simulink model "Group30_SFWR_Assignment1_SIMULINK"  (R2022a)
settings: Solver=FixedStepAuto  StartTime=0.0  StopTime=10  FixedStep=1e-3  RelTol=1e-3  EnableMultiTasking=on
undefined symbols (not defined in the file): D0, D1, D10, D11, D12, D13, D2, D3, D4, D5, D6, D7, D8, D9, PTA0, PTA1, PTA2, PTB23, PTB9, PTC16, PTC17, PTC2, PTC3, PTC4, PTD0, PTD1, PTD2, PTD3
libraries: frdmk64flib x17, etargetslib x2
settings Model: ExtModeTrigDuration=5  Creator=ramu7  LastModifiedBy=scoob
settings OptimizationCC: EnhancedBackFolding=on  PassReuseOutputArgsAs=Individual arguments  ZeroExternalMemoryAtStartup=off  ZeroInternalMemoryAtStartup=off  MaxStackSize=64  OptimizeBlockOrder=speed  DifferentSizesBufferReuse=on  OptimizationCustomize=off  EfficientTunableParamExpr=on
settings DebuggingCC: ParameterTunabilityLossMsg=error
settings HardwareCC: ProdBitPerPointer=32  ProdBitPerSizeT=32  ProdBitPerPtrDiffT=32  ProdLargestAtomicInteger=Long  ProdLargestAtomicFloat=Double  ProdWordSize=32  ProdHWDeviceType=ARM Compatible->ARM Cortex
settings SFSimCC: MATLABDynamicMemAlloc=off
settings RTWCC: SystemTargetFile=ert.tlc  HardwareBoard=NXP FRDM-K64F  TLCOptions="-aInlineSetEventsForThisBaseRateFcn=TLC_FALSE -aSuppressMultiTaskScheduler=TLC_FALSE  -aRateBasedStepFcn=0"  TemplateMakefile=ert_default_tmf  Toolchain=GNU Tools for ARM Embedded Processors
settings CodeAppCC: ForceParamTrailComments=on  IgnoreCustomStorageClasses=off  OperatorAnnotations=on  SimulinkDataObjDesc=on  SFDataObjDesc=on  InsertBlockDesc=on
settings ERTTargetCC: ExtModeTransport=4  ExtModeMexFile=sendToCommService

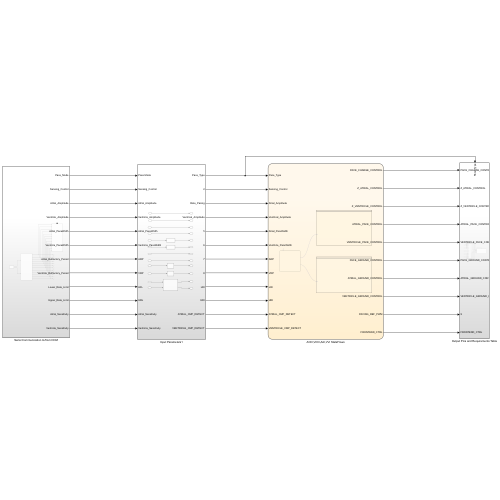
[thumbnail: Simulink's stored preview of the top-level diagram]
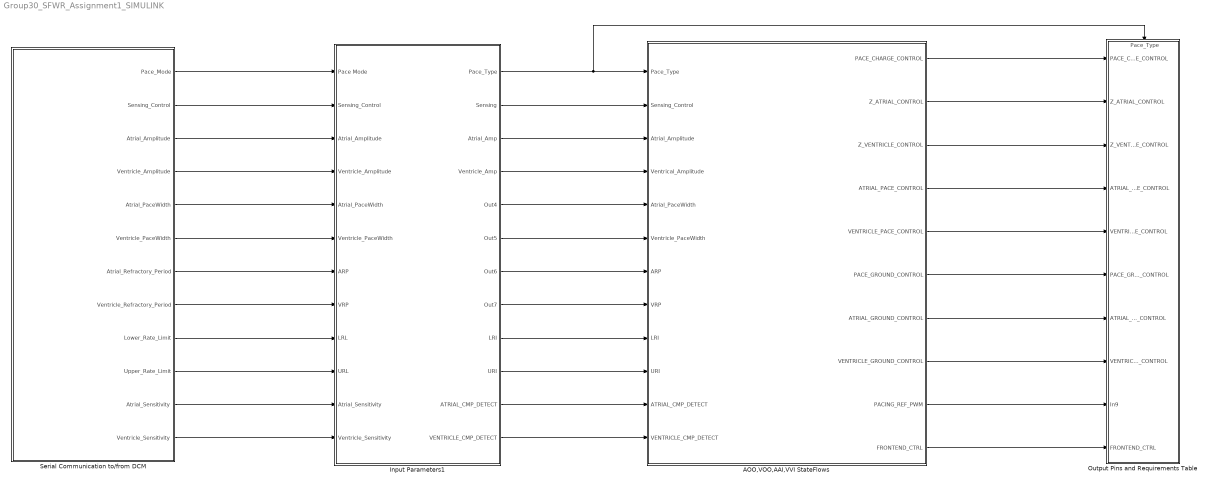
== system Group30_SFWR_Assignment1_SIMULINK ==
  AOO,VOO,AAI,VVI StateFlows : Stateflow chart  TreatAsAtomicUnit=on
      settings: PortSchema="{\"entries\":[{\"content\":{\"sides\":[{\"content\":{\"connectorIds\":[\"In1\",\"In9\",\"In2\",\"In10\",\"In11\",\"In12\",\"In8\",\"In7\",\"In5\",\"In6\",\"In3\",\"In4\"]},\"type\":\"ConnectorPlacement.EquallySpacedRectSide\",\"uuid\":\"9770646f-499d-4715-b3e0-54ec63e9a743\"},{\"content\":{\"connectorIds\":[\"Out1\",\"Out2\",\"Out3\",\"Out4\",\"Out5\",\"Out6\",\"Out7\",\"Out8\",\"Out9\",\"Out10\"],\"side\":\"RIGHT\"},\"type\":\"ConnectorPlacement.EquallySpacedRectSide\",\"uuid\":\"05a40026-c63e-4ef0-b71d-820a20f884f3\"},{\"content\":{\"connectorIds\":[],\"side\":\"TOP\"},\"type\":\"ConnectorPlacement.EquallySpacedRectSide\",\"uuid\":\"87d8712c-6353-4ad8-9661-243ca412d6bb\"}]},\"type\":\"ConnectorPlacement.EquallySpacedConnector\",\"uuid\":\"8262e7ac-98b5-44bf-add5-1ad3a0c707a1\"}],\"packageUris\":[\"http://schema.mathworks.com/mf0/Connector/R2020b\"],\"version\":\"1.0\"}"
  Input Parameters1 : Subsystem
  Output Pins and Requirements Table : Subsystem
      settings: PortSchema="{\"entries\":[{\"content\":{\"sides\":[{\"content\":{\"connectorIds\":[\"In1\",\"In2\",\"In3\",\"In4\",\"In5\",\"In6\",\"In7\",\"In8\",\"In9\",\"In10\"]},\"type\":\"ConnectorPlacement.EquallySpacedRectSide\",\"uuid\":\"40db26f6-8e31-4589-a315-6eea3b6d58f2\"},{\"content\":{\"connectorIds\":[],\"side\":\"RIGHT\"},\"type\":\"ConnectorPlacement.EquallySpacedRectSide\",\"uuid\":\"a6caef76-430e-44a7-94fa-313885a27199\"},{\"content\":{\"connectorIds\":[\"In11\"],\"side\":\"TOP\"},\"type\":\"ConnectorPlacement.EquallySpacedRectSide\",\"uuid\":\"9adbd5f8-a295-4590-a052-0a7aa200e456\"}]},\"type\":\"ConnectorPlacement.EquallySpacedConnector\",\"uuid\":\"6d560563-586d-4d61-8602-6a07324ae70c\"}],\"packageUris\":[\"http://schema.mathworks.com/mf0/Connector/R2020b\"],\"version\":\"1.0\"}"
  Serial Communication to/from DCM : Subsystem
  wires:
  AOO,VOO,AAI,VVI StateFlows/10(FRONTEND_CTRL) -> Output Pins and Requirements Table/10(FRONTEND_CTRL)
  AOO,VOO,AAI,VVI StateFlows/6(PACE_GROUND_CONTROL) -> Output Pins and Requirements Table/6(PACE_GROUND_CONTROL)
  AOO,VOO,AAI,VVI StateFlows/2(Z_ATRIAL_CONTROL) -> Output Pins and Requirements Table/2(Z_ATRIAL_CONTROL)
  AOO,VOO,AAI,VVI StateFlows/3(Z_VENTRICLE_CONTROL) -> Output Pins and Requirements Table/3(Z_VENTRICLE_CONTROL)
  AOO,VOO,AAI,VVI StateFlows/1(PACE_CHARGE_CONTROL) -> Output Pins and Requirements Table/1(PACE_CHARGE_CONTROL)
  AOO,VOO,AAI,VVI StateFlows/4(ATRIAL_PACE_CONTROL) -> Output Pins and Requirements Table/4(ATRIAL_PACE_CONTROL)
  AOO,VOO,AAI,VVI StateFlows/9(PACING_REF_PWM) -> Output Pins and Requirements Table/9(In9)
  AOO,VOO,AAI,VVI StateFlows/7(ATRIAL_GROUND_CONTROL) -> Output Pins and Requirements Table/7(ATRIAL_GROUND_CONTROL)
  AOO,VOO,AAI,VVI StateFlows/5(VENTRICLE_PACE_CONTROL) -> Output Pins and Requirements Table/5(VENTRICLE_PACE_CONTROL)
  AOO,VOO,AAI,VVI StateFlows/8(VENTRICLE_GROUND_CONTROL) -> Output Pins and Requirements Table/8(VENTRICLE_GROUND_CONTROL)
  Input Parameters1/1(Pace_Type) -> Output Pins and Requirements Table/11(Pace_Type), AOO,VOO,AAI,VVI StateFlows/1(Pace_Type)
  Input Parameters1/2(Sensing) -> AOO,VOO,AAI,VVI StateFlows/9(Sensing_Control)
  Input Parameters1/3(Atrial_Amp) -> AOO,VOO,AAI,VVI StateFlows/2(Atrial_Amplitude)
  Input Parameters1/4(Ventricle_Amp) -> AOO,VOO,AAI,VVI StateFlows/10(Ventrical_Amplitude)
  Input Parameters1/6(Out5) -> AOO,VOO,AAI,VVI StateFlows/12(Ventricle_PaceWidth)
  Input Parameters1/5(Out4) -> AOO,VOO,AAI,VVI StateFlows/11(Atrial_PaceWidth)
  Input Parameters1/7(Out6) -> AOO,VOO,AAI,VVI StateFlows/8(ARP)
  Input Parameters1/8(Out7) -> AOO,VOO,AAI,VVI StateFlows/7(VRP)
  Input Parameters1/9(LRI) -> AOO,VOO,AAI,VVI StateFlows/5(LRI)
  Input Parameters1/10(URI) -> AOO,VOO,AAI,VVI StateFlows/6(URI)
  Input Parameters1/11(ATRIAL_CMP_DETECT) -> AOO,VOO,AAI,VVI StateFlows/3(ATRIAL_CMP_DETECT)
  Input Parameters1/12(VENTRICLE_CMP_DETECT) -> AOO,VOO,AAI,VVI StateFlows/4(VENTRICLE_CMP_DETECT)
  Serial Communication to/from DCM/1(Pace_Mode) -> Input Parameters1/1(Pace Mode)
  Serial Communication to/from DCM/2(Sensing_Control) -> Input Parameters1/2(Sensing_Control)
  Serial Communication to/from DCM/3(Atrial_Amplitude) -> Input Parameters1/3(Atrial_Amplitude)
  Serial Communication to/from DCM/4(Ventricle_Amplitude) -> Input Parameters1/4(Ventricle_Amplitude)
  Serial Communication to/from DCM/5(Atrial_PaceWidth) -> Input Parameters1/5(Atrial_PaceWidth)
  Serial Communication to/from DCM/6(Ventricle_PaceWidth) -> Input Parameters1/6(Ventricle_PaceWidth)
  Serial Communication to/from DCM/7(Atrial_Refractory_Period) -> Input Parameters1/7(ARP)
  Serial Communication to/from DCM/8(Ventricle_Refractory_Period) -> Input Parameters1/8(VRP)
  Serial Communication to/from DCM/9(Lower_Rate_Limit) -> Input Parameters1/9(LRL)
  Serial Communication to/from DCM/10(Upper_Rate_Limit) -> Input Parameters1/10(URL)
  Serial Communication to/from DCM/11(Atrial_Sensitivity) -> Input Parameters1/11(Atrial_Sensitivity)
  Serial Communication to/from DCM/12(Ventricle_Sensitivity) -> Input Parameters1/12(Ventricle_Sensitivity)

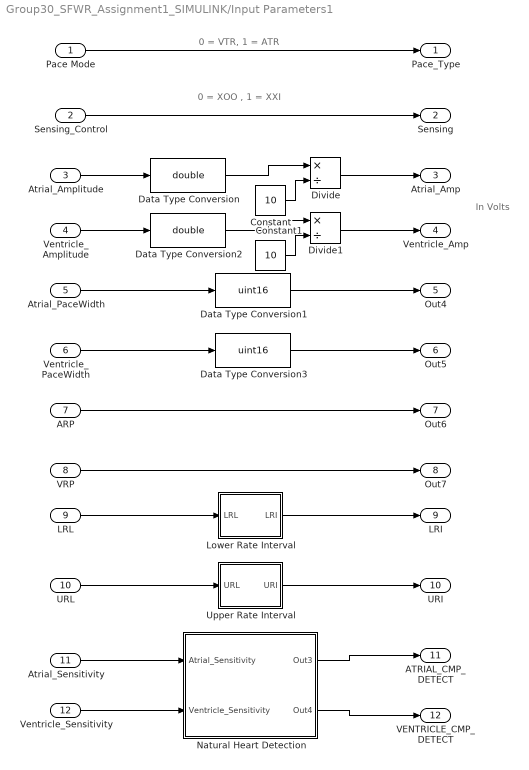
== system Group30_SFWR_Assignment1_SIMULINK/Input Parameters1 ==
  note: In Volts
  note: 0 = XOO , 1 = XXI
  note: 0 = VTR, 1 = ATR
  Pace Mode : Inport  OutDataTypeStr=uint8
  Sensing_Control : Inport  Port=2  OutDataTypeStr=uint8
  Atrial_Amplitude : Inport  Port=3  OutDataTypeStr=uint8
  Ventricle_Amplitude : Inport  Port=4  OutDataTypeStr=uint8
  Atrial_PaceWidth : Inport  Port=5  OutDataTypeStr=uint8
  Ventricle_PaceWidth : Inport  Port=6  OutDataTypeStr=uint8
  ARP : Inport  Port=7  OutDataTypeStr=uint16
  VRP : Inport  Port=8  OutDataTypeStr=uint16
  LRL : Inport  Port=9  OutDataTypeStr=uint8
  URL : Inport  Port=10
  Atrial_Sensitivity : Inport  Port=11  OutDataTypeStr=uint8
  Ventricle_Sensitivity : Inport  Port=12  OutDataTypeStr=uint8
  Constant : Constant  Value=10
  Constant1 : Constant  Value=10
  Data Type Conversion : DataTypeConversion  OutDataTypeStr=double  SaturateOnIntegerOverflow=off  RndMeth=Floor
  Data Type Conversion1 : DataTypeConversion  OutDataTypeStr=uint16  SaturateOnIntegerOverflow=off  RndMeth=Floor
  Data Type Conversion2 : DataTypeConversion  OutDataTypeStr=double  SaturateOnIntegerOverflow=off  RndMeth=Floor
  Data Type Conversion3 : DataTypeConversion  OutDataTypeStr=uint16  SaturateOnIntegerOverflow=off  RndMeth=Floor
  Divide : Product  Inputs=*/
  Divide1 : Product  Inputs=*/
  Lower Rate Interval : Subsystem
  Natural Heart Detection : Subsystem
  Upper Rate Interval : Subsystem
  Pace_Type : Outport
  Sensing : Outport  Port=2
  Atrial_Amp : Outport  Port=3
  Ventricle_Amp : Outport  Port=4
  Out4 : Outport  Port=5
  Out5 : Outport  Port=6
  Out6 : Outport  Port=7
  Out7 : Outport  Port=8
  LRI : Outport  Port=9
  URI : Outport  Port=10
  ATRIAL_CMP_DETECT : Outport  Port=11
  VENTRICLE_CMP_DETECT : Outport  Port=12
  wires:
  Ventricle_PaceWidth/1 -> Data Type Conversion3/1
  VRP/1 -> Out7/1
  Atrial_PaceWidth/1 -> Data Type Conversion1/1
  Sensing_Control/1 -> Sensing/1
  ARP/1 -> Out6/1
  Pace Mode/1 -> Pace_Type/1
  Lower Rate Interval/1(LRI) -> LRI/1
  Upper Rate Interval/1(URI) -> URI/1
  Natural Heart Detection/1(Out3) -> ATRIAL_CMP_DETECT/1
  Natural Heart Detection/2(Out4) -> VENTRICLE_CMP_DETECT/1
  LRL/1 -> Lower Rate Interval/1(LRL)
  URL/1 -> Upper Rate Interval/1(URL)
  Atrial_Sensitivity/1 -> Natural Heart Detection/1(Atrial_Sensitivity)
  Ventricle_Sensitivity/1 -> Natural Heart Detection/2(Ventricle_Sensitivity)
  Data Type Conversion3/1 -> Out5/1
  Data Type Conversion1/1 -> Out4/1
  Atrial_Amplitude/1 -> Data Type Conversion/1
  Data Type Conversion/1 -> Divide/1
  Constant/1 -> Divide/2
  Divide/1 -> Atrial_Amp/1
  Constant1/1 -> Divide1/2
  Data Type Conversion2/1 -> Divide1/1
  Ventricle_Amplitude/1 -> Data Type Conversion2/1
  Divide1/1 -> Ventricle_Amp/1

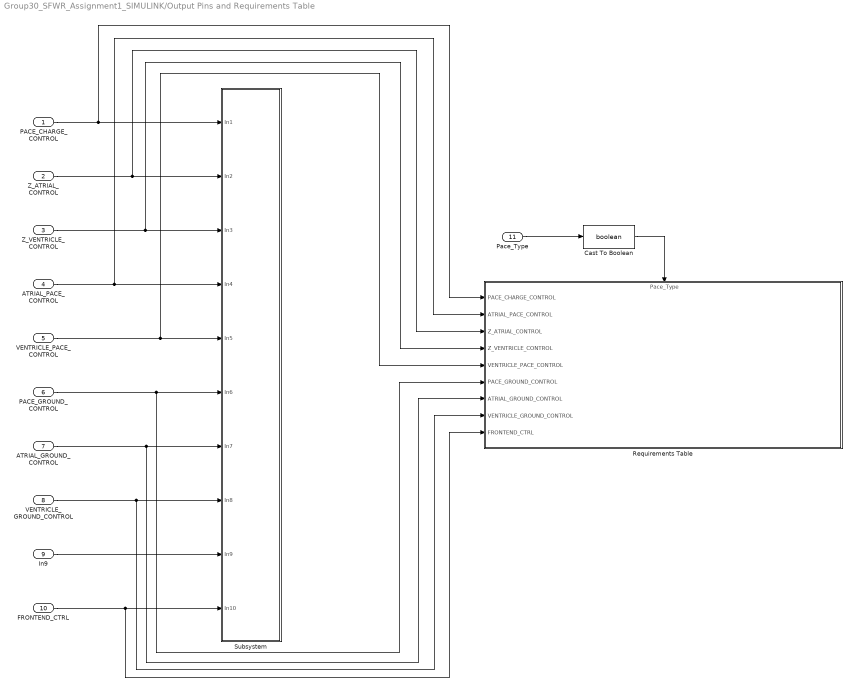
== system Group30_SFWR_Assignment1_SIMULINK/Output Pins and Requirements Table ==
  PACE_CHARGE_CONTROL : Inport
  Z_ATRIAL_CONTROL : Inport  Port=2
  Z_VENTRICLE_CONTROL : Inport  Port=3
  ATRIAL_PACE_CONTROL : Inport  Port=4
  VENTRICLE_PACE_CONTROL : Inport  Port=5
  PACE_GROUND_CONTROL : Inport  Port=6
  ATRIAL_GROUND_CONTROL : Inport  Port=7
  VENTRICLE_GROUND_CONTROL : Inport  Port=8
  In9 : Inport  Port=9
  FRONTEND_CTRL : Inport  Port=10
  Pace_Type : Inport  Port=11
  Cast To Boolean : DataTypeConversion  OutDataTypeStr=boolean  SaturateOnIntegerOverflow=off  RndMeth=Floor
  Requirements Table : Subsystem
      settings: PortSchema="{\"entries\":[{\"content\":{\"sides\":[{\"content\":{\"connectorIds\":[\"In1\",\"In2\",\"In3\",\"In4\",\"In5\",\"In6\",\"In7\",\"In8\",\"In9\"]},\"type\":\"ConnectorPlacement.EquallySpacedRectSide\",\"uuid\":\"46327938-4478-40d2-aac6-72547228615e\"},{\"content\":{\"connectorIds\":[],\"side\":\"RIGHT\"},\"type\":\"ConnectorPlacement.EquallySpacedRectSide\",\"uuid\":\"a4c12f67-beb4-4537-be9d-262931108289\"},{\"content\":{\"connectorIds\":[\"In10\"],\"side\":\"TOP\"},\"type\":\"ConnectorPlacement.EquallySpacedRectSide\",\"uuid\":\"a653f2ff-3266-45dd-85b5-df796fc313fd\"}]},\"type\":\"ConnectorPlacement.EquallySpacedConnector\",\"uuid\":\"ede91063-bb98-4867-a1df-25b64c24a60e\"}],\"packageUris\":[\"http://schema.mathworks.com/mf0/Connector/R2020b\"],\"version\":\"1.0\"}"
  Subsystem : Subsystem
  wires:
  Pace_Type/1 -> Cast To Boolean/1
  PACE_CHARGE_CONTROL/1 -> Requirements Table/1(PACE_CHARGE_CONTROL), Subsystem/1(In1)
  Z_ATRIAL_CONTROL/1 -> Requirements Table/3(Z_ATRIAL_CONTROL), Subsystem/2(In2)
  Z_VENTRICLE_CONTROL/1 -> Requirements Table/4(Z_VENTRICLE_CONTROL), Subsystem/3(In3)
  ATRIAL_PACE_CONTROL/1 -> Requirements Table/2(ATRIAL_PACE_CONTROL), Subsystem/4(In4)
  VENTRICLE_PACE_CONTROL/1 -> Requirements Table/5(VENTRICLE_PACE_CONTROL), Subsystem/5(In5)
  PACE_GROUND_CONTROL/1 -> Requirements Table/6(PACE_GROUND_CONTROL), Subsystem/6(In6)
  ATRIAL_GROUND_CONTROL/1 -> Requirements Table/7(ATRIAL_GROUND_CONTROL), Subsystem/7(In7)
  VENTRICLE_GROUND_CONTROL/1 -> Subsystem/8(In8), Requirements Table/8(VENTRICLE_GROUND_CONTROL)
  In9/1 -> Subsystem/9(In9)
  FRONTEND_CTRL/1 -> Subsystem/10(In10), Requirements Table/9(FRONTEND_CTRL)
  Cast To Boolean/1 -> Requirements Table/10(Pace_Type)

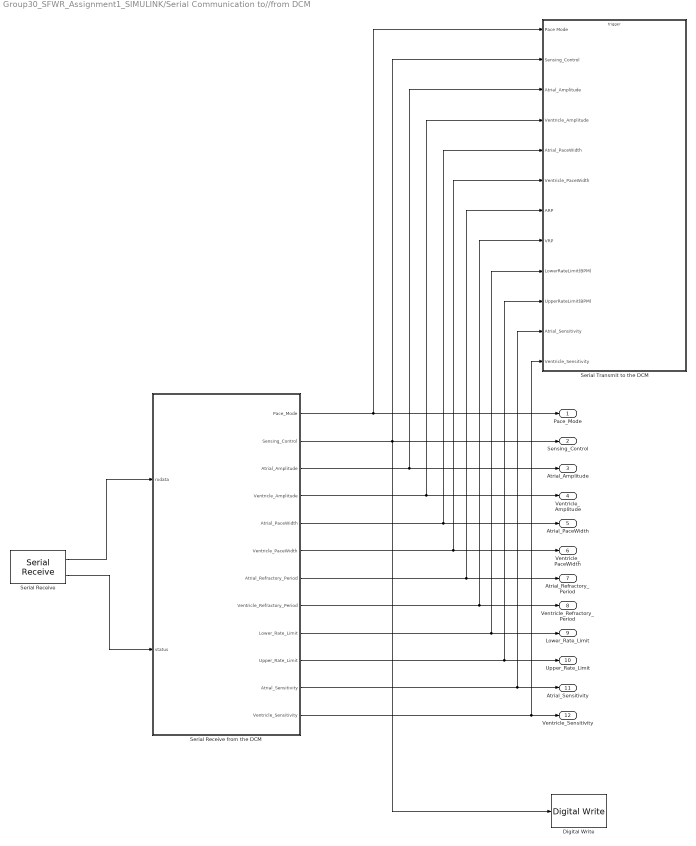
== system Group30_SFWR_Assignment1_SIMULINK/Serial Communication to//from DCM ==
  Digital Write : frdmk64flib/Digital Write  Whichpin=BLUE_LED
  Serial Receive : frdmk64flib/Serial Receive  SCIModule=0  Baudrate=uint32(9600)  Parity=None  StopBits=1  HardwareFlowControl=None  ByteOrder=LittleEndian  DataType=uint8  DataLength=16  BlockingMode=off  OutputStatus=on  SampleTime=-1
  Serial Receive from the DCM : Stateflow chart  TreatAsAtomicUnit=on
      settings: PortSchema="{\"entries\":[{\"content\":{\"sides\":[{\"content\":{\"connectorIds\":[\"In1\",\"In2\"]},\"type\":\"ConnectorPlacement.EquallySpacedRectSide\",\"uuid\":\"2959f4f4-8806-48ae-afb0-f3f6f5a900bd\"},{\"content\":{\"connectorIds\":[\"Out6\",\"Out7\",\"Out1\",\"Out9\",\"Out2\",\"Out10\",\"Out3\",\"Out11\",\"Out5\",\"Out8\",\"Out4\",\"Out12\"],\"side\":\"RIGHT\"},\"type\":\"ConnectorPlacement.EquallySpacedRectSide\",\"uuid\":\"cafcb0cc-74e9-4bf6-9034-07be9eddf5a8\"},{\"content\":{\"connectorIds\":[],\"side\":\"TOP\"},\"type\":\"ConnectorPlacement.EquallySpacedRectSide\",\"uuid\":\"46ea3eb1-522e-47a6-9d77-75fe2cddba2b\"}]},\"type\":\"ConnectorPlacement.EquallySpacedConnector\",\"uuid\":\"dcbaec72-729d-430b-8c38-c6d2009603d6\"}],\"packageUris\":[\"http://schema.mathworks.com/mf0/Connector/R2020b\"],\"version\":\"1.0\"}"
  Serial Transmit to the DCM : Subsystem
  Pace_Mode : Outport
  Sensing_Control : Outport  Port=2
  Atrial_Amplitude : Outport  Port=3
  Ventricle_Amplitude : Outport  Port=4
  Atrial_PaceWidth : Outport  Port=5
  Ventricle_PaceWidth : Outport  Port=6
  Atrial_Refractory_Period : Outport  Port=7
  Ventricle_Refractory_Period : Outport  Port=8
  Lower_Rate_Limit : Outport  Port=9
  Upper_Rate_Limit : Outport  Port=10
  Atrial_Sensitivity : Outport  Port=11
  Ventricle_Sensitivity : Outport  Port=12
  wires:
  Serial Receive from the DCM/8(Upper_Rate_Limit) -> Upper_Rate_Limit/1, Serial Transmit to the DCM/10(UpperRateLimit(BPM))
  Serial Receive from the DCM/11(Ventricle_Refractory_Period) -> Ventricle_Refractory_Period/1, Serial Transmit to the DCM/8(VRP)
  Serial Receive from the DCM/5(Lower_Rate_Limit) -> Lower_Rate_Limit/1, Serial Transmit to the DCM/9(LowerRateLimit(BPM))
  Serial Receive from the DCM/10(Ventricle_PaceWidth) -> Ventricle_PaceWidth/1, Serial Transmit to the DCM/6(Ventricle_PaceWidth)
  Serial Receive from the DCM/6(Pace_Mode) -> Pace_Mode/1, Serial Transmit to the DCM/1(Pace Mode)
  Serial Receive from the DCM/2(Atrial_PaceWidth) -> Atrial_PaceWidth/1, Serial Transmit to the DCM/5(Atrial_PaceWidth)
  Serial Receive from the DCM/4(Atrial_Sensitivity) -> Atrial_Sensitivity/1, Serial Transmit to the DCM/11(Atrial_Sensitivity)
  Serial Receive from the DCM/7(Sensing_Control) -> Digital Write/1, Sensing_Control/1, Serial Transmit to the DCM/2(Sensing_Control)
  Serial Receive from the DCM/1(Atrial_Amplitude) -> Atrial_Amplitude/1, Serial Transmit to the DCM/3(Atrial_Amplitude)
  Serial Receive from the DCM/9(Ventricle_Amplitude) -> Ventricle_Amplitude/1, Serial Transmit to the DCM/4(Ventricle_Amplitude)
  Serial Receive from the DCM/3(Atrial_Refractory_Period) -> Atrial_Refractory_Period/1, Serial Transmit to the DCM/7(ARP)
  Serial Receive from the DCM/12(Ventricle_Sensitivity) -> Ventricle_Sensitivity/1, Serial Transmit to the DCM/12(Ventricle_Sensitivity)
  Serial Receive/1 -> Serial Receive from the DCM/1(rxdata)
  Serial Receive/2 -> Serial Receive from the DCM/2(status)

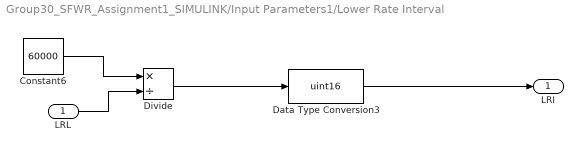
== system Group30_SFWR_Assignment1_SIMULINK/Input Parameters1/Lower Rate Interval ==
  LRL : Inport
  Constant6 : Constant  Value=60000
  Data Type Conversion3 : DataTypeConversion  OutDataTypeStr=uint16  SaturateOnIntegerOverflow=off  RndMeth=Floor
  Divide : Product  Inputs=*/
  LRI : Outport
  wires:
  Constant6/1 -> Divide/1
  LRL/1 -> Divide/2
  Divide/1 -> Data Type Conversion3/1
  Data Type Conversion3/1 -> LRI/1

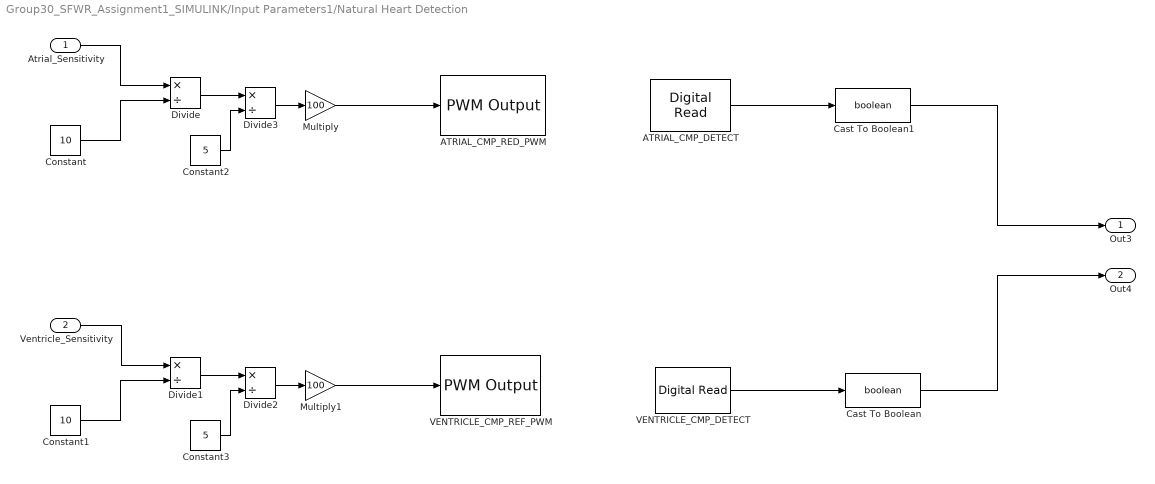
== system Group30_SFWR_Assignment1_SIMULINK/Input Parameters1/Natural Heart Detection ==
  Atrial_Sensitivity : Inport
  Ventricle_Sensitivity : Inport  Port=2
  ATRIAL_CMP_DETECT : frdmk64flib/Digital Read  Whichpin=PTC16 (D0)  SampleTime=-1
  ATRIAL_CMP_RED_PWM : frdmk64flib/PWM Output  Whichpin=PTC2 (D6)  InitialFrequency=2000  InitialDutyCycle=51
  Cast To Boolean : DataTypeConversion  OutDataTypeStr=boolean  SaturateOnIntegerOverflow=off  RndMeth=Floor
  Cast To Boolean1 : DataTypeConversion  OutDataTypeStr=boolean  SaturateOnIntegerOverflow=off  RndMeth=Floor
  Constant : Constant  Value=10
  Constant1 : Constant  Value=10
  Constant2 : Constant  Value=5
  Constant3 : Constant  Value=5
  Divide{,1..3} (4 alike) : Product  Inputs=*/
  Multiply : Gain  Gain=100
  Multiply1 : Gain  Gain=100
  VENTRICLE_CMP_DETECT : frdmk64flib/Digital Read  Whichpin=PTC17 (D1)  SampleTime=-1
  VENTRICLE_CMP_REF_PWM : frdmk64flib/PWM Output  Whichpin=PTA1 (D3)  InitialFrequency=2000  InitialDutyCycle=60
  Out3 : Outport
  Out4 : Outport  Port=2
  wires:
  Multiply1/1 -> VENTRICLE_CMP_REF_PWM/1
  Multiply/1 -> ATRIAL_CMP_RED_PWM/1
  VENTRICLE_CMP_DETECT/1 -> Cast To Boolean/1
  ATRIAL_CMP_DETECT/1 -> Cast To Boolean1/1
  Cast To Boolean1/1 -> Out3/1
  Cast To Boolean/1 -> Out4/1
  Atrial_Sensitivity/1 -> Divide/1
  Constant/1 -> Divide/2
  Constant1/1 -> Divide1/2
  Ventricle_Sensitivity/1 -> Divide1/1
  Divide1/1 -> Divide2/1
  Divide/1 -> Divide3/1
  Constant2/1 -> Divide3/2
  Constant3/1 -> Divide2/2
  Divide3/1 -> Multiply/1
  Divide2/1 -> Multiply1/1

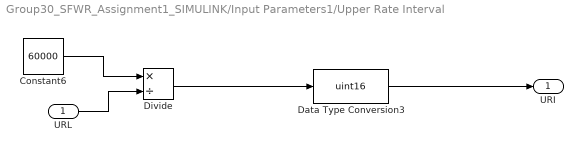
== system Group30_SFWR_Assignment1_SIMULINK/Input Parameters1/Upper Rate Interval ==
  URL : Inport
  Constant6 : Constant  Value=60000
  Data Type Conversion3 : DataTypeConversion  OutDataTypeStr=uint16  SaturateOnIntegerOverflow=off  RndMeth=Floor
  Divide : Product  Inputs=*/
  URI : Outport
  wires:
  Divide/1 -> Data Type Conversion3/1
  URL/1 -> Divide/2
  Constant6/1 -> Divide/1
  Data Type Conversion3/1 -> URI/1

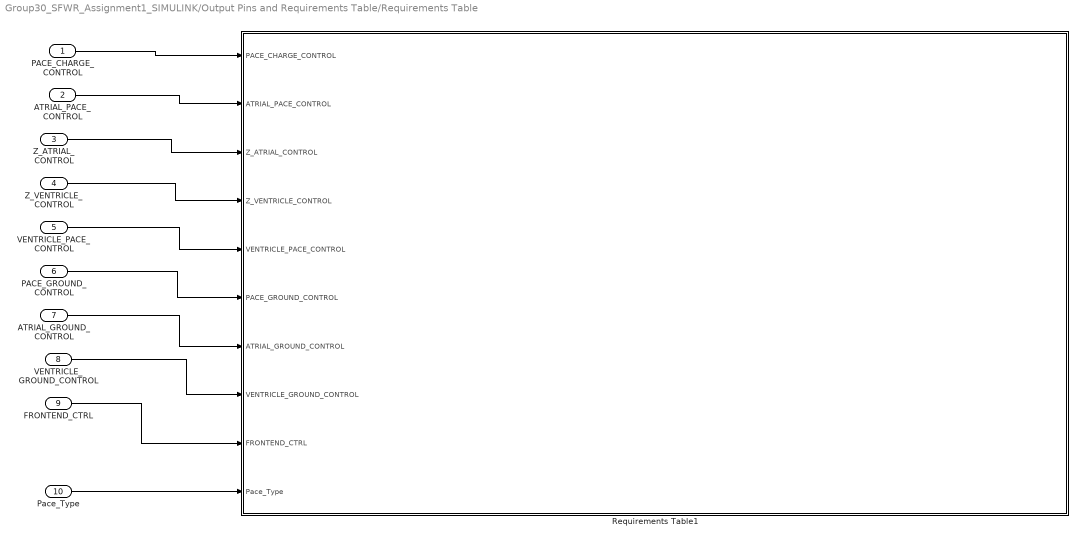
== system Group30_SFWR_Assignment1_SIMULINK/Output Pins and Requirements Table/Requirements Table ==
  PACE_CHARGE_CONTROL : Inport
  ATRIAL_PACE_CONTROL : Inport  Port=2
  Z_ATRIAL_CONTROL : Inport  Port=3
  Z_VENTRICLE_CONTROL : Inport  Port=4
  VENTRICLE_PACE_CONTROL : Inport  Port=5
  PACE_GROUND_CONTROL : Inport  Port=6
  ATRIAL_GROUND_CONTROL : Inport  Port=7
  VENTRICLE_GROUND_CONTROL : Inport  Port=8
  FRONTEND_CTRL : Inport  Port=9
  Pace_Type : Inport  Port=10
  Requirements Table1 : Requirements Table  TreatAsAtomicUnit=on
  wires:
  PACE_CHARGE_CONTROL/1 -> Requirements Table1/1(PACE_CHARGE_CONTROL)
  ATRIAL_PACE_CONTROL/1 -> Requirements Table1/2(ATRIAL_PACE_CONTROL)
  Z_ATRIAL_CONTROL/1 -> Requirements Table1/3(Z_ATRIAL_CONTROL)
  Z_VENTRICLE_CONTROL/1 -> Requirements Table1/4(Z_VENTRICLE_CONTROL)
  VENTRICLE_PACE_CONTROL/1 -> Requirements Table1/5(VENTRICLE_PACE_CONTROL)
  PACE_GROUND_CONTROL/1 -> Requirements Table1/6(PACE_GROUND_CONTROL)
  ATRIAL_GROUND_CONTROL/1 -> Requirements Table1/7(ATRIAL_GROUND_CONTROL)
  VENTRICLE_GROUND_CONTROL/1 -> Requirements Table1/8(VENTRICLE_GROUND_CONTROL)
  FRONTEND_CTRL/1 -> Requirements Table1/9(FRONTEND_CTRL)
  Pace_Type/1 -> Requirements Table1/10(Pace_Type)

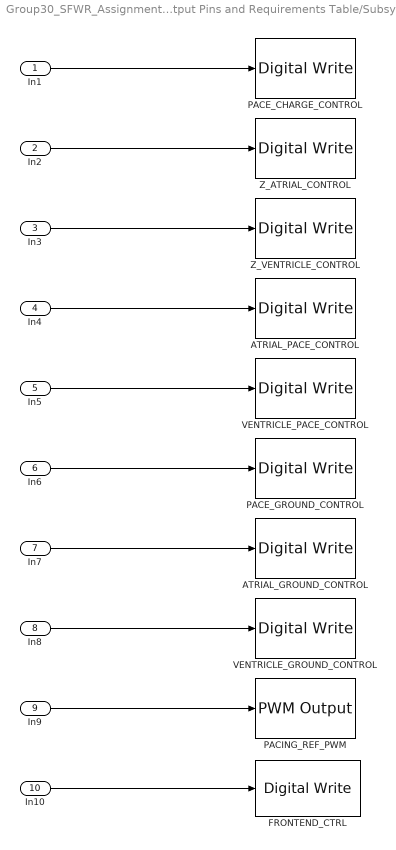
== system Group30_SFWR_Assignment1_SIMULINK/Output Pins and Requirements Table/Subsystem ==
  In1 : Inport
  In2 : Inport  Port=2
  In3 : Inport  Port=3
  In4 : Inport  Port=4
  In5 : Inport  Port=5
  In6 : Inport  Port=6
  In7 : Inport  Port=7
  In8 : Inport  Port=8
  In9 : Inport  Port=9
  In10 : Inport  Port=10
  ATRIAL_GROUND_CONTROL : frdmk64flib/Digital Write  Whichpin=PTD2 (D11)
  ATRIAL_PACE_CONTROL : frdmk64flib/Digital Write  Whichpin=PTA0 (D8)
  FRONTEND_CTRL : frdmk64flib/Digital Write  Whichpin=PTD1 (D13)
  PACE_CHARGE_CONTROL : frdmk64flib/Digital Write  Whichpin=PTB9 (D2)
  PACE_GROUND_CONTROL : frdmk64flib/Digital Write  Whichpin=PTD0 (D10)
  PACING_REF_PWM : frdmk64flib/PWM Output  Whichpin=PTA2 (D5)  InitialFrequency=2000  InitialDutyCycle=40
  VENTRICLE_GROUND_CONTROL : frdmk64flib/Digital Write  Whichpin=PTD3 (D12)
  VENTRICLE_PACE_CONTROL : frdmk64flib/Digital Write  Whichpin=PTC4 (D9)
  Z_ATRIAL_CONTROL : frdmk64flib/Digital Write  Whichpin=PTB23 (D4)
  Z_VENTRICLE_CONTROL : frdmk64flib/Digital Write  Whichpin=PTC3 (D7)
  wires:
  In5/1 -> VENTRICLE_PACE_CONTROL/1
  In9/1 -> PACING_REF_PWM/1
  In7/1 -> ATRIAL_GROUND_CONTROL/1
  In10/1 -> FRONTEND_CTRL/1
  In1/1 -> PACE_CHARGE_CONTROL/1
  In6/1 -> PACE_GROUND_CONTROL/1
  In4/1 -> ATRIAL_PACE_CONTROL/1
  In2/1 -> Z_ATRIAL_CONTROL/1
  In3/1 -> Z_VENTRICLE_CONTROL/1
  In8/1 -> VENTRICLE_GROUND_CONTROL/1

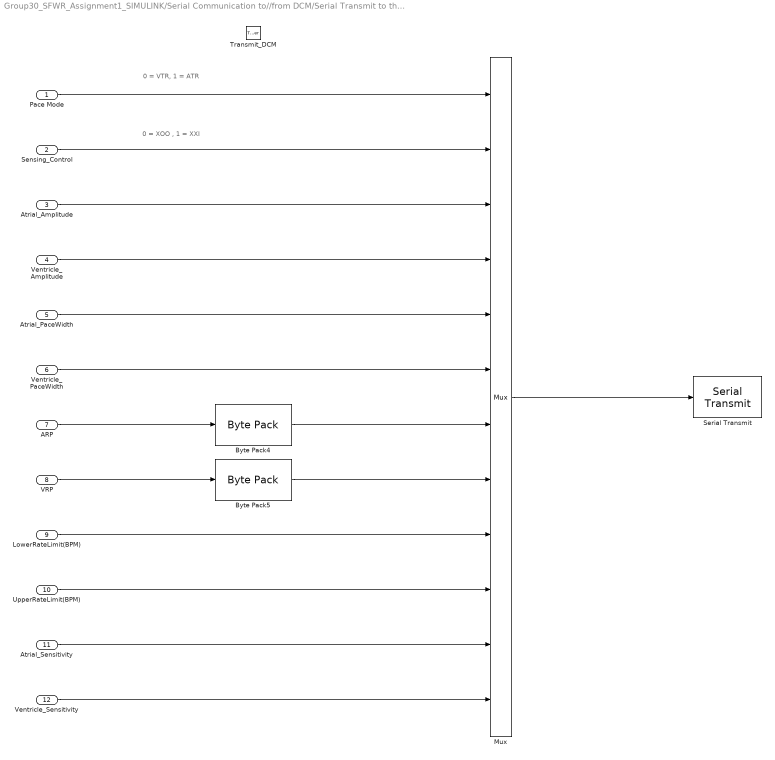
== system Group30_SFWR_Assignment1_SIMULINK/Serial Communication to//from DCM/Serial Transmit to the DCM ==
  note: 0 = VTR, 1 = ATR
  note: 0 = XOO , 1 = XXI
  Pace Mode : Inport  OutDataTypeStr=uint8
  Sensing_Control : Inport  Port=2  OutDataTypeStr=uint8
  Atrial_Amplitude : Inport  Port=3  OutDataTypeStr=uint8
  Ventricle_Amplitude : Inport  Port=4  OutDataTypeStr=uint8
  Atrial_PaceWidth : Inport  Port=5  OutDataTypeStr=uint8
  Ventricle_PaceWidth : Inport  Port=6  OutDataTypeStr=uint8
  ARP : Inport  Port=7  OutDataTypeStr=uint16
  VRP : Inport  Port=8  OutDataTypeStr=uint16
  LowerRateLimit(BPM) : Inport  Port=9
  UpperRateLimit(BPM) : Inport  Port=10
  Atrial_Sensitivity : Inport  Port=11  OutDataTypeStr=uint8
  Ventricle_Sensitivity : Inport  Port=12  OutDataTypeStr=uint8
  Transmit_DCM : TriggerPort  TriggerType=function-call  IsSimulinkFunction=on  FunctionName=Transmit_DCM  VariantControl=Variant
  Byte Pack4 : etargetslib/Byte Pack  datatypes={'uint16'}  byteAlign=1
  Byte Pack5 : etargetslib/Byte Pack  datatypes={'uint16'}  byteAlign=1
  Mux : Mux  Inputs=12
  Serial Transmit : frdmk64flib/Serial Transmit  SCIModule=0  Baudrate=uint32(9600)  Parity=None  StopBits=1  HardwareFlowControl=None  ByteOrder=LittleEndian  BlockingMode=on  OutputStatus=off
  wires:
  Mux/1 -> Serial Transmit/1
  UpperRateLimit(BPM)/1 -> Mux/10
  VRP/1 -> Byte Pack5/1
  ARP/1 -> Byte Pack4/1
  Sensing_Control/1 -> Mux/2
  Pace Mode/1 -> Mux/1
  LowerRateLimit(BPM)/1 -> Mux/9
  Atrial_Amplitude/1 -> Mux/3
  Ventricle_Amplitude/1 -> Mux/4
  Atrial_PaceWidth/1 -> Mux/5
  Ventricle_PaceWidth/1 -> Mux/6
  Byte Pack4/1 -> Mux/7
  Byte Pack5/1 -> Mux/8
  Atrial_Sensitivity/1 -> Mux/11
  Ventricle_Sensitivity/1 -> Mux/12

== stateflow chart Group30_SFWR_Assignment1_SIMULINK/AOO,VOO,AAI,VVI StateFlows ==
  state VENTRICLE MODES (VOO and VVI) [group]
    state SENSE_Ventricle
    note: Heartbeat not found after the LRI period, pace the heart
    note: Heartbeat found, reset LRI
    state PACE_Charge_Ventricle
      %Charging C22 and discharing C21
      entry:
      PACING_REF_PWM = (10*Ventrical_Amplitude/5)
      PACE_CHARGE_CONTROL = true
      VENTRICLE_PACE_CONTROL = false
      VENTRICLE_GROUND_CONTROL=true
      ATRIAL_PACE_CONTROL =false
      ATRIAL_GROUND_CONTROL = false
      FRONTEND_CTRL = false
      PACE_GROUND_CONTROL = true
    state PACE_Discharge_Ventricle
      %Discharging C22
      entry:
      PACE_CHARGE_CONTROL = false
      VENTRICLE_PACE_CONTROL = true
      VENTRICLE_GROUND_CONTROL= false
      FRONTEND_CTRL = false
    SENSE_Ventricle -> PACE_Discharge_Ventricle [order 1] : after(LRI - VRP,msec) [VENTRICLE_CMP_DETECT == false]
    SENSE_Ventricle -> PACE_Charge_Ventricle [order 2] : [VENTRICLE_CMP_DETECT == true]
    PACE_Charge_Ventricle -> SENSE_Ventricle [order 1] : after(VRP,msec)[Sensing_Control == true]{FRONTEND_CTRL = true}
    PACE_Charge_Ventricle -> PACE_Discharge_Ventricle [order 2] : after(LRI - Ventricle_PaceWidth,msec)[Sensing_Control == false]
    PACE_Discharge_Ventricle -> PACE_Charge_Ventricle : after(Ventricle_PaceWidth,msec)
  state Default_State
    entry:
    FRONTEND_CTRL = false
    PACE_GROUND_CONTROL = false
    Z_ATRIAL_CONTROL = false
    Z_VENTRICLE_CONTROL = false
    PACE_CHARGE_CONTROL = false
    VENTRICLE_PACE_CONTROL = false
    VENTRICLE_GROUND_CONTROL = false
    ATRIAL_PACE_CONTROL = false
    ATRIAL_GROUND_CONTROL = false
  state ATRIAL MODES (AOO and AAI) [group]
    state SENSE_Atrial
    note: Heartbeat not found after the LRI period, pace the heart
    note: Heartbeat found, reset LRI
    state PACE_Charge_Atrial
      %Charging C22 and discharing C21
      entry:
      PACING_REF_PWM = (10*Atrial_Amplitude/5)
      PACE_CHARGE_CONTROL = true
      VENTRICLE_PACE_CONTROL = false
      VENTRICLE_GROUND_CONTROL=false
      ATRIAL_PACE_CONTROL =false
      ATRIAL_GROUND_CONTROL = true
      FRONTEND_CTRL = false
      PACE_GROUND_CONTROL = true
    state PACE_Discharge_Atrial
      %Discharging C22
      entry:
      PACE_CHARGE_CONTROL = false
      ATRIAL_PACE_CONTROL = true
      ATRIAL_GROUND_CONTROL = false
      FRONTEND_CTRL = false
    SENSE_Atrial -> PACE_Discharge_Atrial [order 1] : after(LRI - ARP - Atrial_PaceWidth,msec) [ATRIAL_CMP_DETECT == false]
    SENSE_Atrial -> PACE_Charge_Atrial [order 2] : [ATRIAL_CMP_DETECT == true]
    PACE_Charge_Atrial -> SENSE_Atrial [order 1] : after(ARP,msec) [Sensing_Control == true]{FRONTEND_CTRL = true}
    PACE_Charge_Atrial -> PACE_Discharge_Atrial [order 2] : after(LRI - Atrial_PaceWidth,msec)[Sensing_Control == false]
    PACE_Discharge_Atrial -> PACE_Charge_Atrial : after(Atrial_PaceWidth,msec)
  Default_State -> PACE_Charge_Ventricle [order 2] : [Pace_Type == 0]
  (default) -> Default_State
  Default_State -> PACE_Charge_Atrial [order 1] : [Pace_Type == 1]
  data: PACE_CHARGE_CONTROL output; Z_ATRIAL_CONTROL output; Z_VENTRICLE_CONTROL output; ATRIAL_PACE_CONTROL output; VENTRICLE_PACE_CONTROL output; PACE_GROUND_CONTROL output; ATRIAL_GROUND_CONTROL output; VENTRICLE_GROUND_CONTROL output; PACING_REF_PWM output; Pace_Type input uint8; Atrial_Amplitude input uint8; ATRIAL_CMP_DETECT input boolean; VENTRICLE_CMP_DETECT input boolean; LRI input; URI input; VRP input; ARP input; Sensing_Control input uint8; FRONTEND_CTRL output boolean; Ventrical_Amplitude input; Atrial_PaceWidth input; Ventricle_PaceWidth input

== stateflow chart Group30_SFWR_Assignment1_SIMULINK/Serial Communication to//from DCM/Serial Receive from the DCM ==
  settings: executeAtInitialization=1
  state Set_Parameters
    %set the appropriate values based on dcm
    entry:
    Pace_Mode = rxdata(3);
    Sensing_Control = rxdata(4);
    Atrial_Amplitude = rxdata(5); %In (10*Voltage)
    Ventricle_Amplitude = rxdata(6);%In (10*Voltage)
    Atrial_PaceWidth = rxdata(7);%In ms
    Ventricle_PaceWidth = rxdata(8);%In ms
    Atrial_Refractory_Period = typecast(rxdata(9:10),'uint16');%In ms
    Ventricle_Refractory_Period = typecast(rxdata(11:12),'uint16');%In ms
    Lower_Rate_Limit = rxdata(13);%In ppm
    Upper_Rate_Limit = rxdata(14);%In ppm
    Atrial_Sensitivity = rxdata(15);%In (10*Voltage)
    Ventricle_Sensitivity = rxdata(16);%In (10*Voltage)
  state Default_Case
    %Set the initial values of the parameters
    %Nominal Values Used for most cases (some special cases exist)
    entry:
    Pace_Mode = 1;
    Sensing_Control = 0;
    Atrial_Amplitude = 35; %In (10*Voltage)
    Ventricle_Amplitude = 35;%In (10*Voltage)
    Atrial_PaceWidth = 1;%In ms
    Ventricle_PaceWidth = 1;%In ms
    Atrial_Refractory_Period = 250;%In ms
    Ventricle_Refractory_Period = 320;%In ms
    Lower_Rate_Limit = 60;%In ppm
    Upper_Rate_Limit = 120;%In ppm
    Atrial_Sensitivity = 10;%In (10*Voltage)
    Ventricle_Sensitivity = 25;%In (10*Voltage)
  state STANDBY
    %Waiting for COM
  state Echo_Parameters
    entry:
    Transmit_DCM();
  (default) -> Default_Case
  Set_Parameters -> STANDBY
  STANDBY -> (junction 11) : [status == 0]
  (junction 11) -> (junction 16) [order 1] : [rxdata(1)==hex2dec('16')]
  (junction 16) -> Set_Parameters [order 1] : [rxdata(2)==hex2dec('55')]
  Default_Case -> STANDBY
  (junction 11) -> STANDBY [order 2]
  (junction 16) -> Echo_Parameters [order 2] : [rxdata(2)==hex2dec('22')]
  Echo_Parameters -> STANDBY
  data: rxdata input uint8; status input uint8; Atrial_Amplitude output uint8; Atrial_PaceWidth output uint8; Atrial_Refractory_Period output uint16; Atrial_Sensitivity output uint8; Lower_Rate_Limit output uint8; Pace_Mode output uint8; Sensing_Control output uint8; Upper_Rate_Limit output uint8; Ventricle_Amplitude output uint8; Ventricle_PaceWidth output uint8; Ventricle_Refractory_Period output uint16; Ventricle_Sensitivity output uint8

== stateflow chart Group30_SFWR_Assignment1_SIMULINK/Output Pins and Requirements Table/Requirements Table/Requirements Table1 ==
  (default) -> (junction 1073748152)
  (junction 1073748152) -> (junction 1073748153) : {
      | % SF_REQ_REV_07
      | }
  (junction 1073748153) -> (junction 1073748155) : {
      | % HEADER_ASSIGNMENTS
      |
      | }
  (junction 1073748155) -> (junction 1073748157) : {
      | % START_A_4
      | }
  (junction 1073748157) -> (junction 1073748159) : {
      | }
  (junction 1073748159) -> (junction 1073748161)
  (junction 1073748161) -> (junction 1073748163) : {
      | }
  (junction 1073748163) -> (junction 1073748165) : {
      | % END_A_4
      | }
  (junction 1073748165) -> (junction 1073748167) : {
      | % START_R_1
      | }
  (junction 1073748167) -> (junction 1073748169) : {
      | }
  (junction 1073748169) -> (junction 1073748171)
  (junction 1073748171) -> (junction 1073748173) [order 1] : [(((FRONTEND_CTRL) == (1))) && (((PACE_GROUND_CONTROL) == (1))) && (((Pace_Type) == (1)))]
  (junction 1073748171) -> (junction 1073748179) [order 2]
  (junction 1073748173) -> (junction 1073748175) : {
      | reqtable_postcondition((((VENTRICLE_PACE_CONTROL) == (0))) && (((VENTRICLE_GROUND_CONTROL) == (0))) && (((Z_VENTRICLE_CONTROL) == (0))) && (((ATRIAL_PACE_CONTROL) == (0))) && (((ATRIAL_GROUND_CONTROL) == (1))) && (((Z_ATRIAL_CONTROL) == (0))), 'R:1');
      |
      |
      | }
  (junction 1073748175) -> (junction 1073748177) : {
      | }
  (junction 1073748177) -> (junction 1073748179)
  (junction 1073748179) -> (junction 1073748181)
  (junction 1073748181) -> (junction 1073748183) : {
      | % END_R_1
      | }
  (junction 1073748183) -> (junction 1073748185) : {
      | % START_R_19
      | }
  (junction 1073748185) -> (junction 1073748187) : {
      | }
  (junction 1073748187) -> (junction 1073748189)
  (junction 1073748189) -> (junction 1073748191) [order 1] : [(((FRONTEND_CTRL) == (0))) && (((PACE_GROUND_CONTROL) == (1))) && (((Pace_Type) == (1))) && (((PACE_CHARGE_CONTROL) == (0)))]
  (junction 1073748189) -> (junction 1073748197) [order 2]
  (junction 1073748191) -> (junction 1073748193) : {
      | reqtable_postcondition((((VENTRICLE_PACE_CONTROL) == (0))) && (((VENTRICLE_GROUND_CONTROL) == (0))) && (((Z_VENTRICLE_CONTROL) == (0))) && (((ATRIAL_PACE_CONTROL) == (1))) && (((ATRIAL_GROUND_CONTROL) == (0))) && (((Z_ATRIAL_CONTROL) == (0))), 'R:2');
      |
      |
      | }
  (junction 1073748193) -> (junction 1073748195) : {
      | }
  (junction 1073748195) -> (junction 1073748197)
  (junction 1073748197) -> (junction 1073748199)
  (junction 1073748199) -> (junction 1073748201) : {
      | % END_R_19
      | }
  (junction 1073748201) -> (junction 1073748203) : {
      | % START_R_16
      | }
  (junction 1073748203) -> (junction 1073748205) : {
      | }
  (junction 1073748205) -> (junction 1073748207)
  (junction 1073748207) -> (junction 1073748209) [order 1] : [(((FRONTEND_CTRL) == (0))) && (((PACE_GROUND_CONTROL) == (1))) && (((Pace_Type) == (1))) && (((PACE_CHARGE_CONTROL) == (1)))]
  (junction 1073748207) -> (junction 1073748215) [order 2]
  (junction 1073748209) -> (junction 1073748211) : {
      | reqtable_postcondition((((VENTRICLE_PACE_CONTROL) == (0))) && (((VENTRICLE_GROUND_CONTROL) == (0))) && (((Z_VENTRICLE_CONTROL) == (0))) && (((ATRIAL_PACE_CONTROL) == (0))) && (((ATRIAL_GROUND_CONTROL) == (1))) && (((Z_ATRIAL_CONTROL) == (0))), 'R:3');
      |
      |
      | }
  (junction 1073748211) -> (junction 1073748213) : {
      | }
  (junction 1073748213) -> (junction 1073748215)
  (junction 1073748215) -> (junction 1073748217)
  (junction 1073748217) -> (junction 1073748239) : {
      | % END_R_16
      | }
  (junction 1073748239) -> (junction 1073748241) : {
      | % START_R_13
      | }
  (junction 1073748241) -> (junction 1073748243) : {
      | }
  (junction 1073748243) -> (junction 1073748245)
  (junction 1073748245) -> (junction 1073748247) [order 1] : [(((FRONTEND_CTRL) == (1))) && (((PACE_GROUND_CONTROL) == (1))) && (((Pace_Type) == (0)))]
  (junction 1073748245) -> (junction 1073748253) [order 2]
  (junction 1073748247) -> (junction 1073748249) : {
      | reqtable_postcondition((((VENTRICLE_PACE_CONTROL) == (0))) && (((VENTRICLE_GROUND_CONTROL) == (1))) && (((Z_VENTRICLE_CONTROL) == (0))) && (((ATRIAL_PACE_CONTROL) == (0))) && (((ATRIAL_GROUND_CONTROL) == (0))) && (((Z_ATRIAL_CONTROL) == (0))), 'R:4');
      |
      |
      | }
  (junction 1073748249) -> (junction 1073748251) : {
      | }
  (junction 1073748251) -> (junction 1073748253)
  (junction 1073748253) -> (junction 1073748255)
  (junction 1073748255) -> (junction 1073748257) : {
      | % END_R_13
      | }
  (junction 1073748257) -> (junction 1073748259) : {
      | % START_R_10
      | }
  (junction 1073748259) -> (junction 1073748261) : {
      | }
  (junction 1073748261) -> (junction 1073748263)
  (junction 1073748263) -> (junction 1073748265) [order 1] : [(((FRONTEND_CTRL) == (0))) && (((PACE_GROUND_CONTROL) == (1))) && (((Pace_Type) == (0))) && (((PACE_CHARGE_CONTROL) == (0)))]
  (junction 1073748263) -> (junction 1073748271) [order 2]
  (junction 1073748265) -> (junction 1073748267) : {
      | reqtable_postcondition((((VENTRICLE_PACE_CONTROL) == (1))) && (((VENTRICLE_GROUND_CONTROL) == (0))) && (((Z_VENTRICLE_CONTROL) == (0))) && (((ATRIAL_PACE_CONTROL) == (0))) && (((ATRIAL_GROUND_CONTROL) == (0))) && (((Z_ATRIAL_CONTROL) == (0))), 'R:5');
      |
      |
      | }
  (junction 1073748267) -> (junction 1073748269) : {
      | }
  (junction 1073748269) -> (junction 1073748271)
  (junction 1073748271) -> (junction 1073748273)
  (junction 1073748273) -> (junction 1073748275) : {
      | % END_R_10
      | }
  (junction 1073748275) -> (junction 1073748277) : {
      | % START_R_7
      | }
  (junction 1073748277) -> (junction 1073748279) : {
      | }
  (junction 1073748279) -> (junction 1073748281)
  (junction 1073748281) -> (junction 1073748283) [order 1] : [(((FRONTEND_CTRL) == (0))) && (((PACE_GROUND_CONTROL) == (1))) && (((Pace_Type) == (0))) && (((PACE_CHARGE_CONTROL) == (1)))]
  (junction 1073748281) -> (junction 1073748289) [order 2]
  (junction 1073748283) -> (junction 1073748285) : {
      | reqtable_postcondition((((VENTRICLE_PACE_CONTROL) == (0))) && (((VENTRICLE_GROUND_CONTROL) == (1))) && (((Z_VENTRICLE_CONTROL) == (0))) && (((ATRIAL_PACE_CONTROL) == (0))) && (((ATRIAL_GROUND_CONTROL) == (0))) && (((Z_ATRIAL_CONTROL) == (0))), 'R:6');
      |
      |
      | }
  (junction 1073748285) -> (junction 1073748287) : {
      | }
  (junction 1073748287) -> (junction 1073748289)
  (junction 1073748289) -> (junction 1073748291)
  (junction 1073748291) -> (junction 1073748313) : {
      | % END_R_7
      | }
  (junction 1073748313) -> (junction 1073748315) : {
      | % START_R_22
      | }
  (junction 1073748315) -> (junction 1073748317) : {
      | }
  (junction 1073748317) -> (junction 1073748319)
  (junction 1073748319) -> (junction 1073748321) [order 1] : [(((FRONTEND_CTRL) == (0))) && (((PACE_GROUND_CONTROL) == (0))) && (((PACE_CHARGE_CONTROL) == (0)))]
  (junction 1073748319) -> (junction 1073748327) [order 2]
  (junction 1073748321) -> (junction 1073748323) : {
      | reqtable_postcondition((((VENTRICLE_PACE_CONTROL) == (0))) && (((VENTRICLE_GROUND_CONTROL) == (0))) && (((Z_VENTRICLE_CONTROL) == (0))) && (((ATRIAL_PACE_CONTROL) == (0))) && (((ATRIAL_GROUND_CONTROL) == (0))) && (((Z_ATRIAL_CONTROL) == (0))), 'R:7');
      |
      |
      | }
  (junction 1073748323) -> (junction 1073748325) : {
      | }
  (junction 1073748325) -> (junction 1073748327)
  (junction 1073748327) -> (junction 1073748329)
  (junction 1073748329) -> (junction 1073748331) : {
      | % END_R_22
      | }
  data: PACE_CHARGE_CONTROL input boolean; ATRIAL_PACE_CONTROL input boolean; Z_ATRIAL_CONTROL input boolean; Z_VENTRICLE_CONTROL input boolean; VENTRICLE_PACE_CONTROL input boolean; PACE_GROUND_CONTROL input boolean; ATRIAL_GROUND_CONTROL input boolean; VENTRICLE_GROUND_CONTROL input boolean; FRONTEND_CTRL input boolean; Pace_Type input boolean
